simulink model "q11"  (Simulink 8.4)
settings: Solver=ode45  StartTime=0.0  StopTime=10  RelTol=1e-3
settings Model: Creator=didichi  LastModifiedBy=didichi
settings DataIOCC: SignalLoggingSaveFormat=Dataset
settings OptimizationCC: ExpressionDepthLimit=128
settings DebuggingCC: UnderspecifiedInitializationDetection=Simplified  MergeDetectMultiDrivingBlocksExec=error  FcnCallInpInsideContextMsg=EnableAllAsError  StateNameClashWarn=none
settings GRTTargetCC: CombineOutputUpdateFcns=on  GRTInterface=off

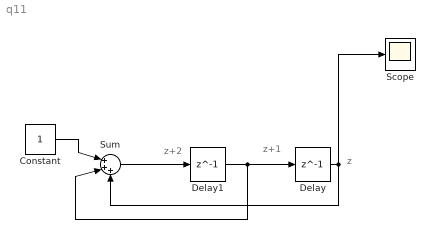
== system q11 ==
  note: z
  note: z+1
  note: z+2
  Constant : Constant
  Delay : Delay  DelayLength=1  SampleTime=1
  Delay1 : Delay  DelayLength=1  SampleTime=1
  Scope : Scope
  Sum : Sum  Inputs=|+++
  wires:
  Sum/1 -> Delay1/1
  Delay1/1 -> Delay/1, Sum/2
  Delay/1 -> Sum/3, Scope/1
  Constant/1 -> Sum/1
